simulink model "ACC_Plant"  (R2025b)
settings: Solver=ode4  StartTime=0.0  StopTime=30.0  FixedStep=0.01  RelTol=1e-3
libraries: simulink x2
Description:
  | Vehicle plant model for Adaptive Cruise Control. Contains longitudinal dynamics of ego vehicle and lead vehicle. Outputs relative distance (d_rel), relative velocity (delta_v), and individual vehicle states for use by ACC controller.
settings Model: Creator=ghazal  LastModifiedBy=ghazal

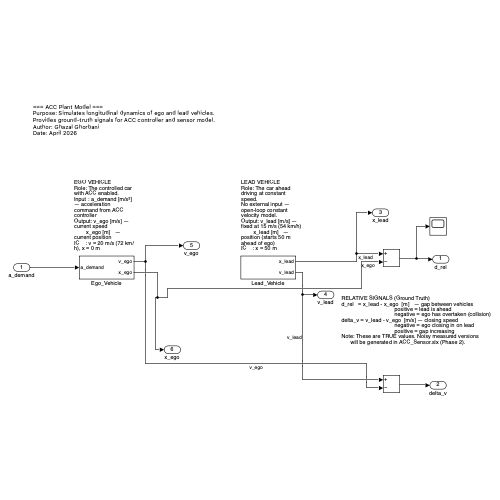
[thumbnail: Simulink's stored preview of the top-level diagram]
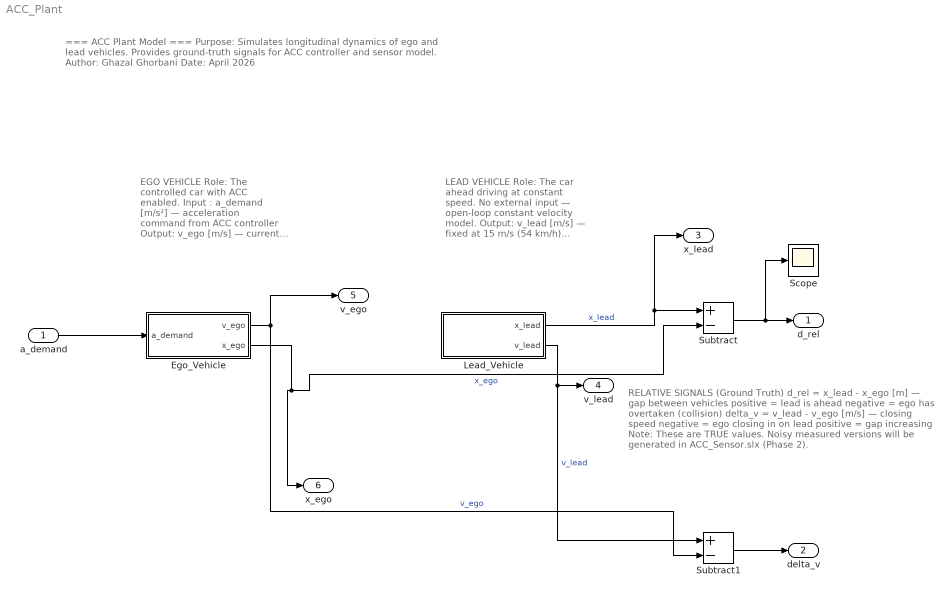
== system ACC_Plant ==
  note: RELATIVE SIGNALS (Ground Truth)
      | d_rel   = x_lead - x_ego  [m]   — gap between vehicles
      |                                    positive = lead is ahead
      |                                    negative = ego has overtaken (collision)
      | delta_v = v_lead - v_ego  [m/s] — closing speed
      |                                    negative = ego closing in on lead
      |                                    positive = gap increasing
      | Note: These are TRUE values. Noisy measured versions
      |       will be generated in ACC_Sensor.slx (Phase 2).
  note: LEAD VEHICLE
      | Role: The car ahead driving at constant speed.
      | No external input — open-loop constant velocity model.
      | Output: v_lead [m/s] — fixed at 15 m/s (54 km/h)
      |         x_lead [m]   — position (starts 50 m ahead of ego)
      | IC    : x = 50 m
  note: === ACC Plant Model ===
      | Purpose: Simulates longitudinal dynamics of ego and lead vehicles.
      | Provides ground-truth signals for ACC controller and sensor model.
      | Author: Ghazal Ghorbani
      | Date: April 2026
  note: EGO VEHICLE
      | Role: The controlled car with ACC enabled.
      | Input : a_demand [m/s²] — acceleration command from ACC controller
      | Output: v_ego [m/s] — current speed
      | x_ego [m] — current position
      | IC : v = 20 m/s (72 km/h), x = 0 m
  a_demand : Inport
  Ego_Vehicle : Subsystem
  Lead_Vehicle : Subsystem
  Scope : Scope
      settings: ActiveDisplayYMinimum=-118.75000000003294  ActiveDisplayYMaximum=68.750000000003652
  Subtract : Sum  Inputs=+-
  Subtract1 : Sum  Inputs=+-
  d_rel : Outport
  delta_v : Outport  Port=2
  x_lead : Outport  Port=3
  v_lead : Outport  Port=4
  v_ego : Outport  Port=5
  x_ego : Outport  Port=6
  wires:
  Lead_Vehicle/1(x_lead) -> x_lead/1, Subtract/1  "x_lead"
  Ego_Vehicle/2(x_ego) -> Subtract/2, x_ego/1  "x_ego"
  Subtract/1 -> Scope/1, d_rel/1
  Lead_Vehicle/2(v_lead) -> v_lead/1, Subtract1/1  "v_lead"
  Ego_Vehicle/1(v_ego) -> Subtract1/2, v_ego/1  "v_ego"
  Subtract1/1 -> delta_v/1
  a_demand/1 -> Ego_Vehicle/1(a_demand)

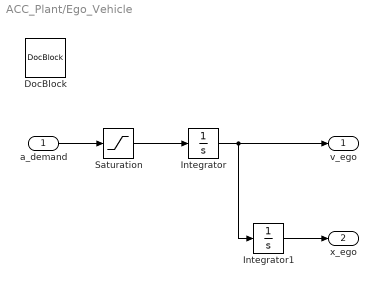
== system ACC_Plant/Ego_Vehicle ==
  a_demand : Inport
  DocBlock : simulink/Model-Wide Utilities/DocBlock  DocumentType=Text
      content=|
      | SUBSYSTEM: Ego_Vehicle
      | ========================================
      | DESCRIPTION:
      |   Models the longitudinal dynamics of the ego vehicle
      |   (the car equipped with ACC) on a straight highway.
      |   Assumes flat road, no aerodynamic drag (simplified model).
      |
      | SIGNAL FLOW:
      |   a_demand → Saturation → Integrator(v) → Integrator(x)
      |
      | PARAMETERS:
      |   Saturation upper limit : +3  m/s²
      |     Rationale: Typical comfortable max acceleration for a passenger car.
      |
      |   Saturation lower limit : -8  m/s²
      |     Rationale: Hard braking limit (approx. 0.8g).
      |                Emergency brake in real ACC is ~-5 to -8 m/s².
      |
      |   Integrator 1 (a → v_ego):
      |     Initial condition : 20 m/s
      |     Rationale: Ego starts at highway speed (72 km/h).
      |                Lead vehicle is at 15 m/s → gap closes immediately
      |                without controller, confirming plant is correct.
      |
      |   Integrator 2 (v_ego → x_ego):
      |     Initial condition : 0 m
      |     Rationale: Ego defined as origin. Lead starts at +50 m.
      |
      | INPUTS:
      |   a_demand  [m/s²]  Acceleration demand from ACC controller
      |                     (will be connected in Phase 4)
      |
      | OUTPUTS:
      |   v_ego  [m/s]  Ego vehicle longitudinal speed
      |   x_ego  [m]   Ego vehicle longitudinal position
      |
      | ASSUMPTIONS:
      |   - 1D longitudinal motion only (no lateral dynamics)
      |   - Flat road (no gradient)
      |   - Vehicle mass effects abstracted into acceleration demand
      |   - Tire slip and actuator delays not modelled (future work)
      |
      | VALIDATION:
      |   With a_demand = 0: v_ego constant at 20 m/s. ✓
      |   d_rel decreases at -5 m/s slope over 30s. ✓
  Integrator : Integrator  InitialCondition=20
  Integrator1 : Integrator
  Saturation : Saturate  UpperLimit=3  LowerLimit=-8
  v_ego : Outport
  x_ego : Outport  Port=2
  wires:
  a_demand/1 -> Saturation/1
  Integrator/1 -> Integrator1/1, v_ego/1
  Saturation/1 -> Integrator/1
  Integrator1/1 -> x_ego/1

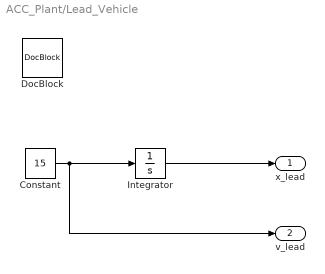
== system ACC_Plant/Lead_Vehicle ==
  Constant : Constant  Value=15
  DocBlock : simulink/Model-Wide Utilities/DocBlock  DocumentType=Text
      content=|
      | SUBSYSTEM: Lead_Vehicle
      | ========================================
      | DESCRIPTION:
      |   Models the lead vehicle (the car ahead of the ego vehicle).
      |   Simplified open-loop model: constant speed, no driver input.
      |   In Phase 6 this will be replaced with a dynamic profile
      |   to simulate braking, cut-in and cut-out scenarios.
      |
      | SIGNAL FLOW:
      |   Constant(v_lead) → Integrator(x_lead)
      |   Constant(v_lead) ─────────────────────→ output port v_lead
      |
      | PARAMETERS:
      |   Constant speed : 15 m/s (54 km/h)
      |     Rationale: Slower than ego (20 m/s) to create a closing
      |                scenario that tests ACC follow mode immediately.
      |
      |   Integrator (v_lead → x_lead):
      |     Initial condition : 50 m
      |     Rationale: Lead vehicle starts 50 m ahead of ego.
      |                Represents a realistic highway following scenario.
      |                Minimum safe following distance at 20 m/s with
      |                t_gap = 2.5s would be ~50 m, so initial gap
      |                is at the boundary — intentional stress test.
      |
      | OUTPUTS:
      |   x_lead  [m]   Lead vehicle longitudinal position
      |   v_lead  [m/s] Lead vehicle longitudinal speed (constant)
      |
      | FUTURE WORK (Phase 6):
      |   Replace Constant block with Signal Builder or MATLAB Function
      |   to implement:
      |     - Scenario A: Lead vehicle braking at t=10s
      |     - Scenario B: Cut-in vehicle at close range
      |     - Scenario C: Lead vehicle accelerating away
  Integrator : Integrator  InitialCondition=50
  x_lead : Outport
  v_lead : Outport  Port=2
  wires:
  Integrator/1 -> x_lead/1
  Constant/1 -> v_lead/1, Integrator/1
